simulink model "ERR_H5"  (R2025a)
settings: Solver=VariableStepAuto  StartTime=0.0  StopTime=5  MaxStep=100e-3/25  RelTol=1e-3
libraries: simulink_extras x1
settings Model: Creator=Szalay  LastModifiedBy=Szalay

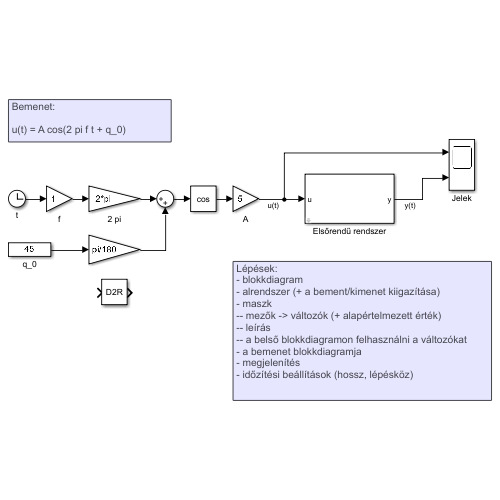
[thumbnail: Simulink's stored preview of the top-level diagram]
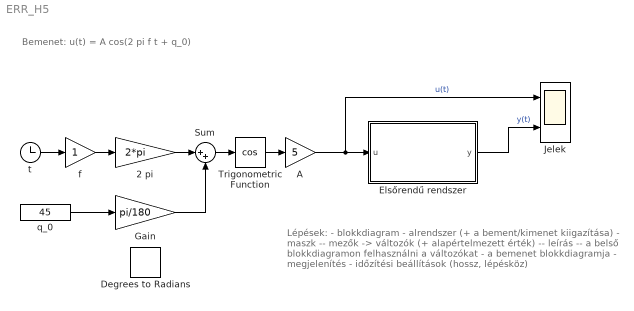
== system ERR_H5 ==
  note: Lépések:
      | - blokkdiagram
      | - alrendszer (+ a bement/kimenet kiigazítása)
      | - maszk
      | -- mezők -> változók (+ alapértelmezett érték)
      | -- leírás
      | -- a belső blokkdiagramon felhasználni a változókat
      | - a bemenet blokkdiagramja
      | - megjelenítés
      | - időzítési beállítások (hossz, lépésköz)
  note: Bemenet:
      |
      | u(t) = A cos(2 pi f t + q_0)
  2 pi : Gain  Gain=2*pi
  A : Gain  Gain=5
  Degrees to Radians : simulink_extras/Transformations/Degrees to Radians
  Elsőrendű rendszer : Subsystem  mask(Elsőrendű rendszer){y_0=0, K=1, tau=1}
      mask prompts: y_0 "Kezdeti érték"; K "Állandósult állapoti erősítés"; tau "Időállandó (s)"
      mask help: A lineáris elsőrendű rendszer modellje.
      mask DialogControl ParameterGroupVar Prompt: Modellparaméterek
      mask DialogControl Container3 Prompt: Kezdeti érték
  Gain : Gain  Gain=pi/180
  Jelek : Scope  NumInputPorts=2
      settings: ActiveDisplayYMinimum=-6.2498109071402759  ActiveDisplayYMaximum=6.2498109071402768
  Sum : Sum  Inputs=|++
  Trigonometric Function : Trigonometry  Operator=cos
  f : Gain
  q_0 : Constant  Value=45
  t : Clock
  wires:
  A/1 -> Jelek/1, Elsőrendű rendszer/1(u)  "u(t)"
  Trigonometric Function/1 -> A/1
  Sum/1 -> Trigonometric Function/1
  q_0/1 -> Gain/1
  Gain/1 -> Sum/2
  t/1 -> f/1
  2 pi/1 -> Sum/1
  f/1 -> 2 pi/1
  Elsőrendű rendszer/1(y) -> Jelek/2  "y(t)"

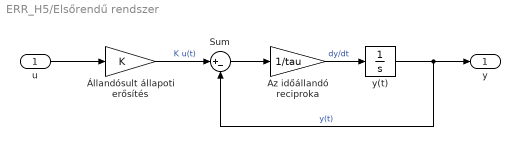
== system ERR_H5/Elsőrendű rendszer ==
  u : Inport
  Az időállandó reciproka : Gain  Gain=1/tau
  Sum : Sum  Inputs=|+-
  y(t) : Integrator  InitialCondition=y_0
  Állandósult állapoti erősítés : Gain  Gain=K
  y : Outport
  wires:
  Az időállandó reciproka/1 -> y(t)/1  "dy/dt"
  Állandósult állapoti erősítés/1 -> Sum/1  "K u(t)"
  Sum/1 -> Az időállandó reciproka/1
  y(t)/1 -> y/1, Sum/2  "y(t)"
  u/1 -> Állandósult állapoti erősítés/1
